simulink model "ttNCM_Wrapper"  (Simulink 7.3)
settings: Solver=ode45  StartTime=0.0  StopTime=10.0  RelTol=1e-3
undefined symbols (not defined in the file or in its folder): ttNCM
settings Model: Creator=Ayush Gupta  LastModifiedBy=Ayush Gupta

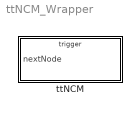
== system ttNCM_Wrapper ==
  ttNCM : Subsystem  mask(ttNCM Wrapper){nNbr=1}
      mask prompts: nNbr "networkNbr"
      mask help: Specify the Network Number

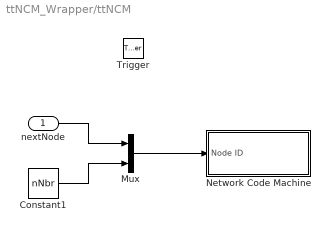
== system ttNCM_Wrapper/ttNCM ==
  nextNode : Inport  OutDataType=fixdt(1, 16)  OutScaling=2^0
  Trigger : TriggerPort  TriggerType=either
  Constant1 : Constant  Value=nNbr  OutDataType=fixdt(1, 16)  OutScaling=2^0
  Mux : Mux  Inputs=2
  Network Code Machine : Subsystem  AncestorBlock=NCM/Network Code Machine  TreatAsAtomicUnit=on
  wires:
  nextNode/1 -> Mux/1
  Constant1/1 -> Mux/2
  Mux/1 -> Network Code Machine/1(Node ID)

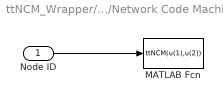
== system ttNCM_Wrapper/ttNCM/Network Code Machine ==
  Node ID : Inport
  MATLAB Fcn : MATLABFcn  MATLABFcn=ttNCM(u(1),u(2))  OutputDimensions=0
  wires:
  Node ID/1 -> MATLAB Fcn/1
